simulink model "Buck_Direct_SMC"  (R2021a)
settings: Solver=VariableStepAuto  StartTime=0.0  StopTime=0.01  RelTol=1e-7
libraries: spsSeriesRLCBranchLib x3, spsDiodeLib x3, spsCurrentMeasurementLib x2, spsDCVoltageSourceLib x1, spsIdealSwitchLib x1, spsVoltageMeasurementLib x1, spspowerguiLib x1
settings Model: Creator=Asus  LastModifiedBy=rapha
settings DebuggingCC: UnconnectedInputMsg=none  UnconnectedOutputMsg=none  UnconnectedLineMsg=none
settings ModelReferenceCC: EnableRefExpFcnMdlSchedulingChecks=off
settings RTWCC: Description=Generic Real-Time Target  DLArmComputeVersion=20.02.1

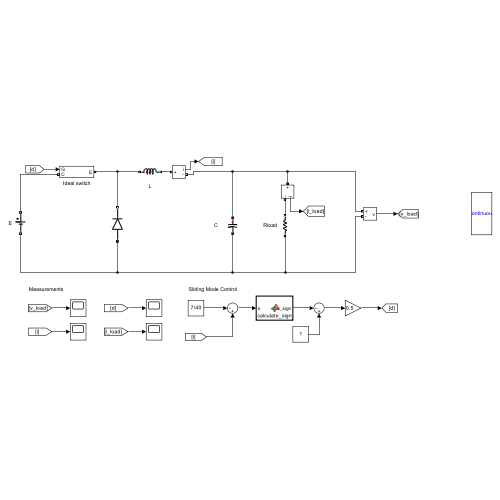
[thumbnail: Simulink's stored preview of the top-level diagram]
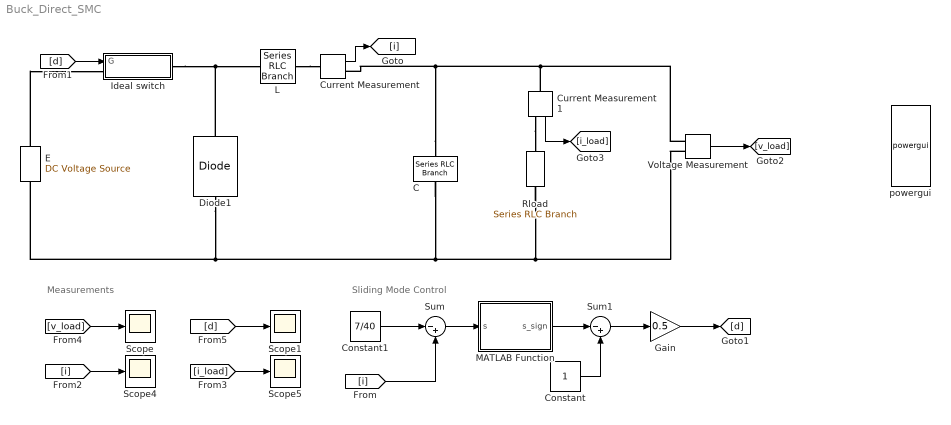
== system Buck_Direct_SMC ==
  note: Measurements
  note: Sliding Mode Control
  C : spsSeriesRLCBranchLib/Series RLC Branch  LConnTagsString=__new0  RConnTagsString=__new0  BranchType=C  Resistance=1  Inductance=1e-3  SetiL0=off  InitialCurrent=0  Capacitance=0.000004  Setx0=off  InitialVoltage=0  Measurements=None
  Constant : Constant
  Constant1 : Constant  Value=7/40
  Current Measurement : spsCurrentMeasurementLib/Current Measurement  PhasorSimulation=off  OutputType=Complex  PSBequivalent=0
  Current Measurement1 : spsCurrentMeasurementLib/Current Measurement  PhasorSimulation=off  OutputType=Complex  PSBequivalent=0
  Diode1 : spsDiodeLib/Diode  Ron=0.001  Lon=0  Vf=0  IC=0  UseSnubber=0  Rs=inf  Cs=inf  Measurements=off
  E : spsDCVoltageSourceLib/DC Voltage Source  Amplitude=20  Measurements=None
  Gain : Gain  Gain=0.5
  Ideal switch : Subsystem
  L : spsSeriesRLCBranchLib/Series RLC Branch  LConnTagsString=__new0  RConnTagsString=__new0  BranchType=L  Resistance=1  Inductance=0.040  SetiL0=off  InitialCurrent=0  Capacitance=1e-6  Setx0=off  InitialVoltage=0  Measurements=None
  MATLAB Function : MATLAB Function  TreatAsAtomicUnit=on
  Rload : spsSeriesRLCBranchLib/Series RLC Branch  LConnTagsString=__new0  RConnTagsString=__new0  BranchType=R  Resistance=40  Inductance=1e-3  SetiL0=off  InitialCurrent=0  Capacitance=1e-6  Setx0=off  InitialVoltage=0  Measurements=None
  Scope{,1,4..5} (4 alike) : Scope
  Sum : Sum  Inputs=|-+
  Sum1 : Sum  Inputs=|-+
  Voltage Measurement : spsVoltageMeasurementLib/Voltage Measurement  PhasorSimulation=off  OutputType=Complex  PSBequivalent=0
  powergui : spspowerguiLib/powergui  Priority=1  SimulationMode=Continuous  SampleTime=1/20000000  frequency=60  Iterations=50  frequencyindice=0  Pbase=100e6  ErrMax=1e-4  UnitsV=kV  UnitsW=MW  buscounter=0  FunctionMessages=off  echomessages=off  EnableUseOfTLC=off  CurrentSourceSwitches=off  DisableSnubberDevices=off  DisableRonSwitches=off  DisableVfSwitches=off  DisplayEquations=off  AutomaticDiscreteSolvers=off  SolverType=Tustin/Backward Euler (TBE)  Interpol=off  ExternalGateDelay=off  methode=off  Ts=100  x0status=blocks  SPID=on  SwTol=0  HookPort=off  NonlinearTolerance=1e-4  nMaxIteration=100  ContinueOnMaxIteration=off  RestoreLinks=warning  ResistiveCurrentMeasurement=off  Frange=[0:2:500]  Ylog=off  Xlog=on  ShowGrid=off  save=off  variable=ZData  structure=0  ZoomFFT=off  StartTime=0.0  cycles=1  DisplayStyle=1  fundamental=60  FreqAxis=off  MaxFrequency=1000  frequencyindicesteady=1  RmsSteady=1  display=off
  wires:
  Current Measurement/1 -> [i]
  [d] -> Ideal switch/1(G)
  Voltage Measurement/1 -> [v_load]
  Current Measurement1/1 -> [i_load]
  [v_load] -> Scope/1
  [i] -> Scope4/1
  [i_load] -> Scope5/1
  [d] -> Scope1/1
  [i] -> Sum/2
  Sum/1 -> MATLAB Function/1(s)
  Gain/1 -> [d]
  MATLAB Function/1(s_sign) -> Sum1/1
  Constant1/1 -> Sum/1
  Constant/1 -> Sum1/2
  Sum1/1 -> Gain/1
  connections:
  Rload/RConn1 -- Voltage Measurement/LConn2 -- C/RConn1 -- Diode1/LConn1 -- E/LConn1
  E/RConn1 -- Ideal switch/LConn1
  Ideal switch/RConn1 -- Diode1/RConn1 -- L/LConn1
  L/RConn1 -- Current Measurement/LConn1
  C/LConn1 -- Current Measurement1/LConn1 -- Voltage Measurement/LConn1 -- Current Measurement/RConn1
  Current Measurement1/RConn1 -- Rload/LConn1

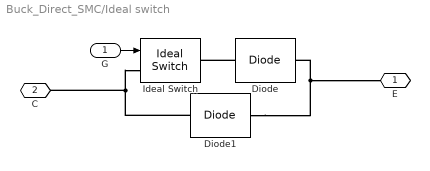
== system Buck_Direct_SMC/Ideal switch ==
  G : Inport
  Diode : spsDiodeLib/Diode  Ron=0  Lon=0  Vf=0  IC=0  UseSnubber=0  Rs=inf  Cs=inf  Measurements=off
  Diode1 : spsDiodeLib/Diode  Ron=0  Lon=0  Vf=0  IC=0  UseSnubber=0  Rs=inf  Cs=inf  Measurements=off
  Ideal Switch : spsIdealSwitchLib/Ideal Switch  Ron=0  Lon=0  IC=1  Rs=inf  Cs=inf  Measurements=off
  E : PMIOPort  Side=Right
  C : PMIOPort  Port=2  Side=Left
  wires:
  G/1 -> Ideal Switch/1
  connections:
  Diode/LConn1 -- Ideal Switch/RConn1
  Diode1/RConn1 -- Ideal Switch/LConn1 -- C/RConn1
  Diode1/LConn1 -- E/RConn1 -- Diode/RConn1

== matlab function Buck_Direct_SMC/MATLAB Function ==
  data: s input; s_sign output
function s_sign = calculate_sign(s)

if(s > 0)
    s_sign = 1;
elseif (s == 0)
    s_sign = 0;
else 
    s_sign = -1;
end
return
